simulink model "PMSM_Drehstrom_Regelung"  (R2014b)
settings: Solver=ode4  StartTime=0.0  StopTime=5  FixedStep=1e-6  RelTol=1e-3
undefined symbols (not defined in the file): J, Ld, Lq, n_soll, p, Psi_pm, R1
libraries: simulink x2
settings Model: Creator=benjamin  LastModifiedBy=Benji

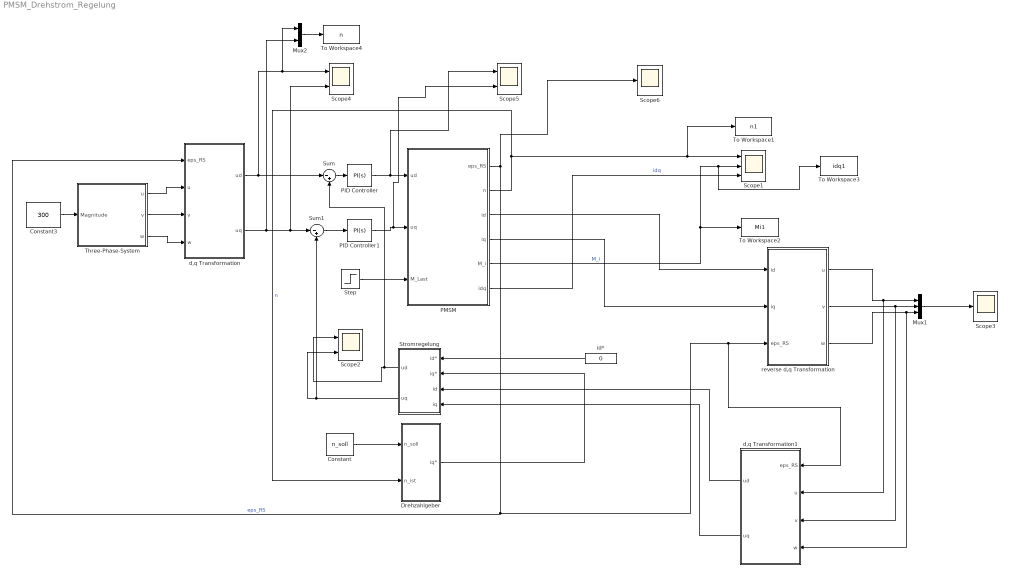
== system PMSM_Drehstrom_Regelung ==
  Constant : Constant  Value=n_soll
  Constant3 : Constant  Value=300
  Drehzahlgeber : Subsystem
  Mux1 : Mux  Inputs=3
  Mux2 : Mux  Inputs=2
  PID Controller : simulink/Continuous/PID Controller  Controller=PI  TimeDomain=Continuous-time  SampleTime=-1  IntegratorMethod=Forward Euler  FilterMethod=Forward Euler  Form=Parallel  P=10  I=1  D=0  N=100  InitialConditionSource=internal  InitialConditionForIntegrator=0  InitialConditionForFilter=0  ExternalReset=none  LimitOutput=off  UpperSaturationLimit=inf  LowerSaturationLimit=-inf  LinearizeAsGain=on  AntiWindupMode=none  Kb=1  TrackingMode=off  Kt=1  PParamMin=[]  PParamMax=[]  IParamMin=[]  IParamMax=[]  DParamMin=[]  DParamMax=[]  NParamMin=[]  NParamMax=[]  KbParamMin=[]  KbParamMax=[]  KtParamMin=[]  KtParamMax=[]  POutMin=[]  POutMax=[]  IOutMin=[]  IOutMax=[]  DOutMin=[]  DOutMax=[]  NOutMin=[]  NOutMax=[]  KbOutMin=[]  KbOutMax=[]  KtOutMin=[]  KtOutMax=[]  IntegratorOutMin=[]  IntegratorOutMax=[]  FilterOutMin=[]  FilterOutMax=[]  SumOutMin=[]  SumOutMax=[]  SumI1OutMin=[]  SumI1OutMax=[]  SumI2OutMin=[]  SumI2OutMax=[]  SumI3OutMin=[]  SumI3OutMax=[]  SumDOutMin=[]  SumDOutMax=[]  SaturationOutMin=[]  SaturationOutMax=[]  IntegratorContinuousStateAttributes=''  IntegratorStateMustResolveToSignalObject=off  IntegratorRTWStateStorageClass=Auto  FilterContinuousStateAttributes=''  FilterStateMustResolveToSignalObject=off  FilterRTWStateStorageClass=Auto  DifferentiatorICPrevScaledInput=0  DifferentiatorOutMin=[]  DifferentiatorOutMax=[]  UseFilter=on
  PID Controller1 : simulink/Continuous/PID Controller  Controller=PI  TimeDomain=Continuous-time  SampleTime=-1  IntegratorMethod=Forward Euler  FilterMethod=Forward Euler  Form=Parallel  P=10  I=1  D=0  N=100  InitialConditionSource=internal  InitialConditionForIntegrator=0  InitialConditionForFilter=0  ExternalReset=none  LimitOutput=off  UpperSaturationLimit=inf  LowerSaturationLimit=-inf  LinearizeAsGain=on  AntiWindupMode=none  Kb=1  TrackingMode=off  Kt=1  PParamMin=[]  PParamMax=[]  IParamMin=[]  IParamMax=[]  DParamMin=[]  DParamMax=[]  NParamMin=[]  NParamMax=[]  KbParamMin=[]  KbParamMax=[]  KtParamMin=[]  KtParamMax=[]  POutMin=[]  POutMax=[]  IOutMin=[]  IOutMax=[]  DOutMin=[]  DOutMax=[]  NOutMin=[]  NOutMax=[]  KbOutMin=[]  KbOutMax=[]  KtOutMin=[]  KtOutMax=[]  IntegratorOutMin=[]  IntegratorOutMax=[]  FilterOutMin=[]  FilterOutMax=[]  SumOutMin=[]  SumOutMax=[]  SumI1OutMin=[]  SumI1OutMax=[]  SumI2OutMin=[]  SumI2OutMax=[]  SumI3OutMin=[]  SumI3OutMax=[]  SumDOutMin=[]  SumDOutMax=[]  SaturationOutMin=[]  SaturationOutMax=[]  IntegratorContinuousStateAttributes=''  IntegratorStateMustResolveToSignalObject=off  IntegratorRTWStateStorageClass=Auto  FilterContinuousStateAttributes=''  FilterStateMustResolveToSignalObject=off  FilterRTWStateStorageClass=Auto  DifferentiatorICPrevScaledInput=0  DifferentiatorOutMin=[]  DifferentiatorOutMax=[]  UseFilter=on
  PMSM : Subsystem
  Scope1 : Scope  NumInputPorts=3
      settings: TimeRange=0.112043795620438  YMin=0~-1000~-4000  YMax=5000~2500~6000  SaveName=ScopeData3
  Scope2 : Scope  NumInputPorts=2
      settings: TimeRange=0.2  YMin=-25000~-400  YMax=20000~400  SaveName=ScopeData2
  Scope3 : Scope
      settings: TimeRange=0.02  YMin=0  YMax=5000  SaveName=ScopeData4
  Scope4 : Scope  NumInputPorts=2
      settings: TimeRange=0.2  YMin=-25000~-400  YMax=20000~400  SaveName=ScopeData5
  Scope5 : Scope  NumInputPorts=2
      settings: TimeRange=0.2  YMin=-25000~-400  YMax=20000~400  SaveName=ScopeData6
  Scope6 : Scope
      settings: TimeRange=0.02  YMin=0  YMax=5000  SaveName=ScopeData7
  Step : Step  Time=0.08  After=30  SampleTime=0
  Stromregelung : Subsystem
  Sum : Sum  Inputs=|-+
  Sum1 : Sum  Inputs=|-+
  Three-Phase-System : Subsystem
  To Workspace1 : ToWorkspace  VariableName=n1  SaveFormat=Timeseries  SampleTime=-1
  To Workspace2 : ToWorkspace  VariableName=Mi1  SaveFormat=Timeseries  SampleTime=-1
  To Workspace3 : ToWorkspace  VariableName=idq1  SaveFormat=Timeseries  SampleTime=-1
  To Workspace4 : ToWorkspace  VariableName=n  SaveFormat=Timeseries  SampleTime=-1
  d,q Transformation : Subsystem
  d,q Transformation1 : Subsystem
  id* : Constant  Value=0
  reverse d,q Transformation : Subsystem
  wires:
  id*/1 -> Stromregelung/1(id*)
  Drehzahlgeber/1(iq*) -> Stromregelung/2(iq*)
  Constant/1 -> Drehzahlgeber/1(n_soll)
  PMSM/2(n) -> To Workspace1/1, Scope1/1, Drehzahlgeber/2(n_ist)  "n"
  PMSM/6(idq) -> Scope1/3  "idq"
  Step/1 -> PMSM/3(M_Last)
  Stromregelung/1(ud) -> Sum/2, Scope2/1
  Stromregelung/2(uq) -> Sum1/2, Scope2/2
  Constant3/1 -> Three-Phase-System/1(Magnitude)
  Three-Phase-System/1(u) -> d,q Transformation/2(u)
  Three-Phase-System/2(v) -> d,q Transformation/3(v)
  Three-Phase-System/3(w) -> d,q Transformation/4(w)
  PMSM/1(eps_RS) -> d,q Transformation1/1(eps_RS), reverse d,q Transformation/3(eps_RS), d,q Transformation/1(eps_RS), Scope6/1  "eps_RS"
  PMSM/3(id) -> reverse d,q Transformation/1(id)
  PMSM/4(iq) -> reverse d,q Transformation/2(iq)
  reverse d,q Transformation/1(u) -> d,q Transformation1/2(u), Mux1/1
  reverse d,q Transformation/2(v) -> Mux1/2, d,q Transformation1/3(v)
  reverse d,q Transformation/3(w) -> d,q Transformation1/4(w), Mux1/3
  Mux1/1 -> Scope3/1
  PMSM/5(M_i) -> To Workspace2/1, To Workspace3/1, Scope1/2  "M_i"
  d,q Transformation/1(ud) -> Mux2/1, Scope4/1, Sum/1
  d,q Transformation/2(uq) -> Mux2/2, Scope4/2, Sum1/1
  Sum/1 -> PID Controller/1
  PID Controller/1 -> Scope5/1, PMSM/1("ud ")
  Sum1/1 -> PID Controller1/1
  PID Controller1/1 -> Scope5/2, PMSM/2(uq)
  d,q Transformation1/1(ud) -> Stromregelung/3(id)
  d,q Transformation1/2(uq) -> Stromregelung/4(iq)
  Mux2/1 -> To Workspace4/1

== system PMSM_Drehstrom_Regelung/Drehzahlgeber ==
  n_soll : Inport
  n_ist : Inport  Port=2
  Gain : Gain  Gain=10
  Gain1 : Gain  Gain=2
  Integrator : Integrator
  Sum : Sum  Inputs=|+-
  Sum1 : Sum  Inputs=|++
  iq* : Outport
  wires:
  n_soll/1 -> Sum/1
  n_ist/1 -> Sum/2
  Sum/1 -> Gain1/1, Gain/1
  Gain/1 -> Sum1/1
  Gain1/1 -> Integrator/1
  Integrator/1 -> Sum1/2
  Sum1/1 -> iq*/1

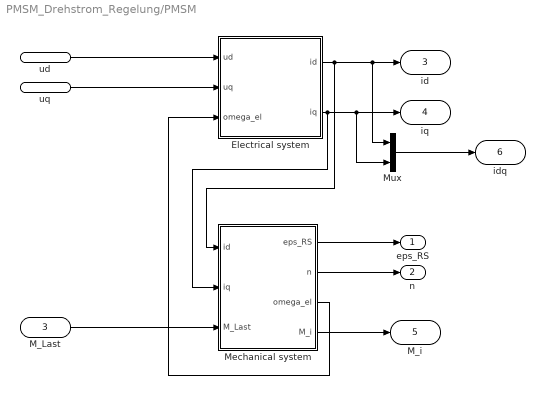
== system PMSM_Drehstrom_Regelung/PMSM ==
  "ud " : Inport
  uq : Inport  Port=2
  M_Last : Inport  Port=3
  Electrical system : Subsystem
  Mechanical system : Subsystem
  Mux : Mux  Inputs=2
  eps_RS : Outport
  n : Outport  Port=2
  id : Outport  Port=3
  iq : Outport  Port=4
  M_i : Outport  Port=5
  idq : Outport  Port=6
  wires:
  Electrical system/1(id) -> Mux/1, id/1, Mechanical system/1(id)
  Electrical system/2(iq) -> Mux/2, iq/1, Mechanical system/2(iq)
  Mechanical system/3(omega_el) -> Electrical system/3(omega_el)
  Mechanical system/1(eps_RS) -> eps_RS/1
  Mechanical system/2(n) -> n/1
  Mechanical system/4(M_i) -> M_i/1
  M_Last/1 -> Mechanical system/3(M_Last)
  uq/1 -> Electrical system/2(uq)
  "ud "/1 -> Electrical system/1(ud)
  Mux/1 -> idq/1

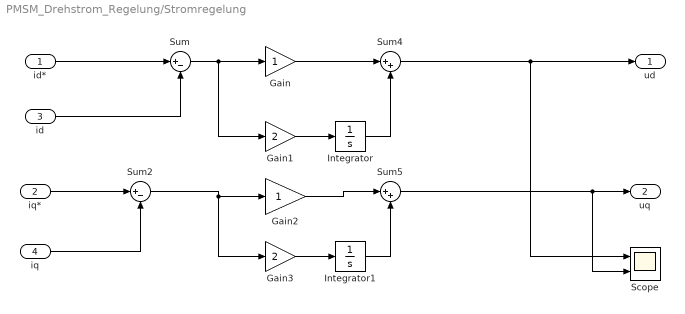
== system PMSM_Drehstrom_Regelung/Stromregelung ==
  id* : Inport
  iq* : Inport  Port=2
  id : Inport  Port=3
  iq : Inport  Port=4
  Gain : Gain
  Gain1 : Gain  Gain=2
  Gain2 : Gain
  Gain3 : Gain  Gain=2
  Integrator : Integrator
  Integrator1 : Integrator
  Scope : Scope  NumInputPorts=2
      settings: TimeRange=5  YMin=-1.3~-5  YMax=0~5
  Sum : Sum  Inputs=|+-
  Sum2 : Sum  Inputs=|+-
  Sum4 : Sum  Inputs=|++
  Sum5 : Sum  Inputs=|++
  ud : Outport
  uq : Outport  Port=2
  wires:
  Sum5/1 -> Scope/2, uq/1
  iq*/1 -> Sum2/1
  id*/1 -> Sum/1
  id/1 -> Sum/2
  iq/1 -> Sum2/2
  Sum4/1 -> ud/1, Scope/1
  Sum/1 -> Gain1/1, Gain/1
  Gain/1 -> Sum4/1
  Gain1/1 -> Integrator/1
  Integrator/1 -> Sum4/2
  Sum2/1 -> Gain3/1, Gain2/1
  Gain2/1 -> Sum5/1
  Gain3/1 -> Integrator1/1
  Integrator1/1 -> Sum5/2

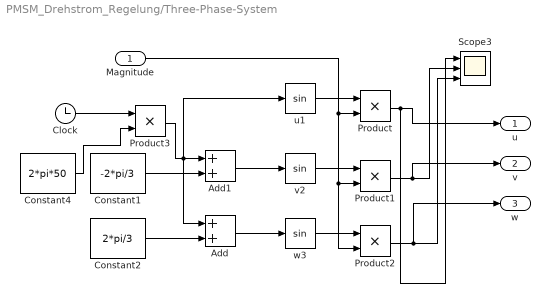
== system PMSM_Drehstrom_Regelung/Three-Phase-System ==
  Magnitude : Inport
  Add : Sum
  Add1 : Sum
  Clock : Clock
  Constant1 : Constant  Value=-2*pi/3
  Constant2 : Constant  Value=2*pi/3
  Constant4 : Constant  Value=2*pi*50
  Product{,1..3} (4 alike) : Product
  Scope3 : Scope  NumInputPorts=3
      settings: YMin=-5~-5~-5  YMax=5~5~5
  u1 : Trigonometry
  v2 : Trigonometry
  w3 : Trigonometry
  u : Outport
  v : Outport  Port=2
  w : Outport  Port=3
  wires:
  Constant2/1 -> Add/2
  Add/1 -> w3/1
  Add1/1 -> v2/1
  Constant1/1 -> Add1/2
  Product2/1 -> w/1, Scope3/3
  Product/1 -> u/1, Scope3/1
  w3/1 -> Product2/1
  Product3/1 -> Add/1, Add1/1, u1/1
  Clock/1 -> Product3/1
  Product1/1 -> v/1, Scope3/2
  Constant4/1 -> Product3/2
  Magnitude/1 -> Product2/2, Product1/2, Product/2
  u1/1 -> Product/1
  v2/1 -> Product1/1

== system PMSM_Drehstrom_Regelung/d,q Transformation ==
  eps_RS : Inport
  u : Inport  Port=2
  v : Inport  Port=3
  w : Inport  Port=4
  Clarke Transformation : Subsystem
  Park Transformation : Subsystem
  ud : Outport
  uq : Outport  Port=2
  wires:
  eps_RS/1 -> Park Transformation/3(epsilonRS)
  Clarke Transformation/1(alpha) -> Park Transformation/1(alpha)
  Clarke Transformation/2(beta) -> Park Transformation/2(beta)
  Park Transformation/1(d) -> ud/1
  Park Transformation/2(q) -> uq/1
  v/1 -> Clarke Transformation/2(v)
  u/1 -> Clarke Transformation/1(u)
  w/1 -> Clarke Transformation/3(w)

== system PMSM_Drehstrom_Regelung/d,q Transformation1 ==
  eps_RS : Inport
  u : Inport  Port=2
  v : Inport  Port=3
  w : Inport  Port=4
  Clarke Transformation : Subsystem
  Park Transformation : Subsystem
  ud : Outport
  uq : Outport  Port=2
  wires:
  eps_RS/1 -> Park Transformation/3(epsilonRS)
  Clarke Transformation/1(alpha) -> Park Transformation/1(alpha)
  Clarke Transformation/2(beta) -> Park Transformation/2(beta)
  Park Transformation/1(d) -> ud/1
  Park Transformation/2(q) -> uq/1
  v/1 -> Clarke Transformation/2(v)
  u/1 -> Clarke Transformation/1(u)
  w/1 -> Clarke Transformation/3(w)

== system PMSM_Drehstrom_Regelung/reverse d,q Transformation ==
  id : Inport
  iq : Inport  Port=2
  eps_RS : Inport  Port=3
  inverse Clarke Transformation : Subsystem
  inverse Park Transformation : Subsystem
  u : Outport
  v : Outport  Port=2
  w : Outport  Port=3
  wires:
  inverse Clarke Transformation/2(iv) -> v/1
  id/1 -> inverse Park Transformation/1(d)
  inverse Clarke Transformation/1(iu) -> u/1
  iq/1 -> inverse Park Transformation/2(q)
  inverse Clarke Transformation/3(iw) -> w/1
  eps_RS/1 -> inverse Park Transformation/3(epsilonRS)
  inverse Park Transformation/1(alpha) -> inverse Clarke Transformation/1(alpha)
  inverse Park Transformation/2(beta) -> inverse Clarke Transformation/2(beta)

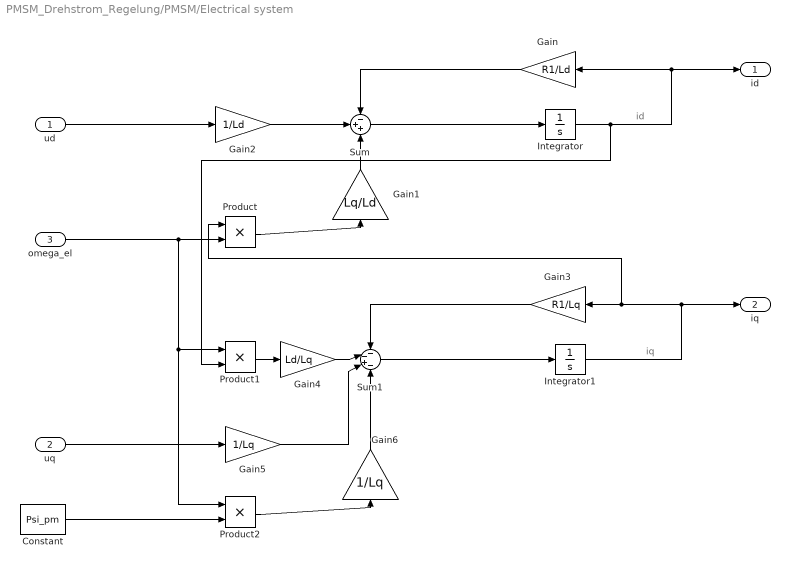
== system PMSM_Drehstrom_Regelung/PMSM/Electrical system ==
  note: id
  note: iq
  ud : Inport
  uq : Inport  Port=2
  omega_el : Inport  Port=3
  Constant : Constant  Value=Psi_pm
  Gain : Gain  Gain=R1/Ld
  Gain1 : Gain  Gain=Lq/Ld
  Gain2 : Gain  Gain=1/Ld
  Gain3 : Gain  Gain=R1/Lq
  Gain4 : Gain  Gain=Ld/Lq
  Gain5 : Gain  Gain=1/Lq
  Gain6 : Gain  Gain=1/Lq
  Integrator : Integrator
  Integrator1 : Integrator
  Product : Product
  Product1 : Product
  Product2 : Product
  Sum : Sum  Inputs=-++
  Sum1 : Sum  Inputs=--+-
  id : Outport
  iq : Outport  Port=2
  wires:
  Sum/1 -> Integrator/1
  Integrator/1 -> Product1/2, Gain/1, id/1
  Gain/1 -> Sum/1
  omega_el/1 -> Product2/1, Product1/1, Product/2
  Gain1/1 -> Sum/3
  Product/1 -> Gain1/1
  ud/1 -> Gain2/1
  Gain2/1 -> Sum/2
  Sum1/1 -> Integrator1/1
  Integrator1/1 -> iq/1, Product/1, Gain3/1
  Gain3/1 -> Sum1/1
  Gain5/1 -> Sum1/3
  Product1/1 -> Gain4/1
  Gain4/1 -> Sum1/2
  uq/1 -> Gain5/1
  Constant/1 -> Product2/2
  Gain6/1 -> Sum1/4
  Product2/1 -> Gain6/1

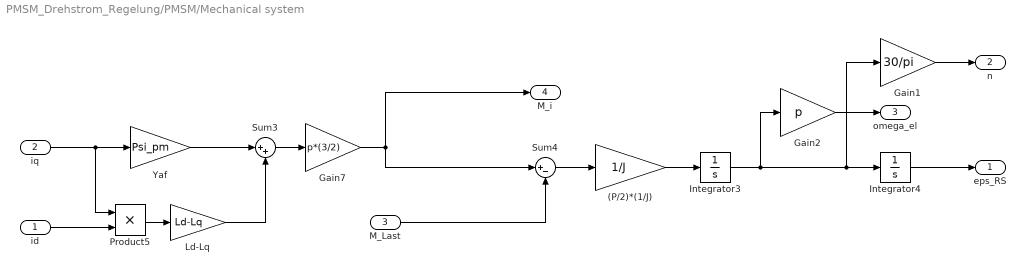
== system PMSM_Drehstrom_Regelung/PMSM/Mechanical system ==
  id : Inport
  iq : Inport  Port=2
  M_Last : Inport  Port=3
  (P/2)*(1/J) : Gain  Gain=1/J
  Gain1 : Gain  Gain=30/pi
  Gain2 : Gain  Gain=p
  Gain7 : Gain  Gain=p*(3/2)
  Integrator3 : Integrator
  Integrator4 : Integrator
  Ld-Lq : Gain  Gain=Ld-Lq
  Product5 : Product  RndMeth=Zero
  Sum3 : Sum  Inputs=|++
  Sum4 : Sum  Inputs=|+-
  Yaf : Gain  Gain=Psi_pm
  eps_RS : Outport
  n : Outport  Port=2
  omega_el : Outport  Port=3
  M_i : Outport  Port=4
  wires:
  Yaf/1 -> Sum3/1
  Sum3/1 -> Gain7/1
  Ld-Lq/1 -> Sum3/2
  Product5/1 -> Ld-Lq/1
  Sum4/1 -> (P/2)*(1/J)/1
  iq/1 -> Product5/1, Yaf/1
  id/1 -> Product5/2
  Gain7/1 -> Sum4/1, M_i/1
  (P/2)*(1/J)/1 -> Integrator3/1
  Integrator4/1 -> eps_RS/1
  Gain1/1 -> n/1
  Integrator3/1 -> Gain1/1, Integrator4/1, Gain2/1
  M_Last/1 -> Sum4/2
  Gain2/1 -> omega_el/1

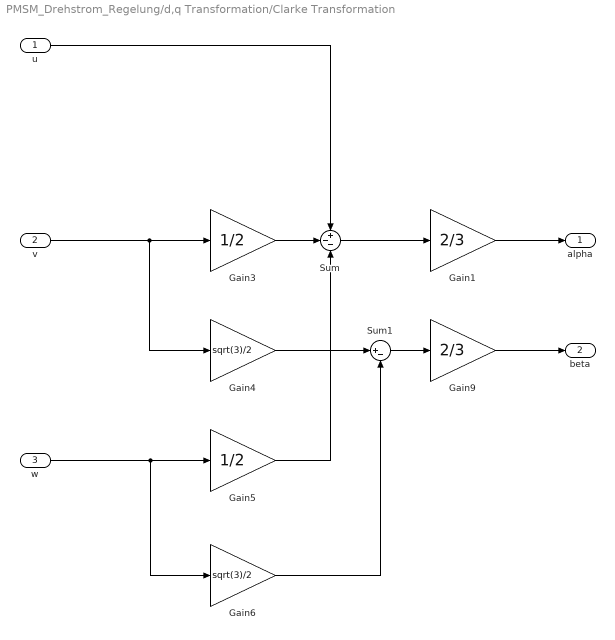
== system PMSM_Drehstrom_Regelung/d,q Transformation/Clarke Transformation ==
  u : Inport
  v : Inport  Port=2
  w : Inport  Port=3
  Gain1 : Gain  Gain=2/3
  Gain3 : Gain  Gain=1/2
  Gain4 : Gain  Gain=sqrt(3)/2
  Gain5 : Gain  Gain=1/2
  Gain6 : Gain  Gain=sqrt(3)/2
  Gain9 : Gain  Gain=2/3
  Sum : Sum  Inputs=+--
  Sum1 : Sum  Inputs=|+-
  alpha : Outport
  beta : Outport  Port=2
  wires:
  Gain5/1 -> Sum/3
  Gain3/1 -> Sum/2
  v/1 -> Gain4/1, Gain3/1
  w/1 -> Gain6/1, Gain5/1
  Gain6/1 -> Sum1/2
  Gain4/1 -> Sum1/1
  Sum/1 -> Gain1/1
  Gain1/1 -> alpha/1
  u/1 -> Sum/1
  Sum1/1 -> Gain9/1
  Gain9/1 -> beta/1

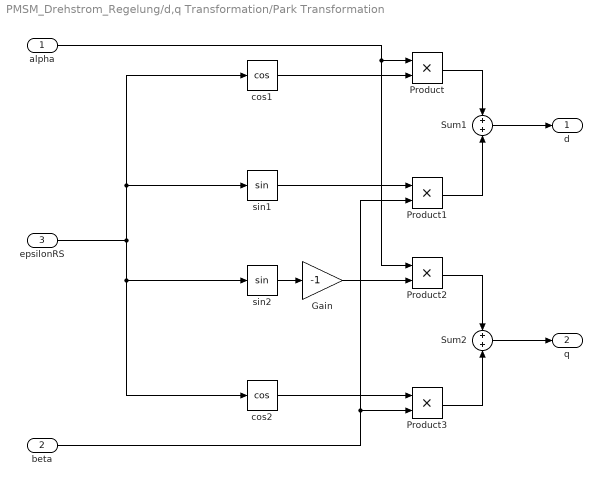
== system PMSM_Drehstrom_Regelung/d,q Transformation/Park Transformation ==
  alpha : Inport
  beta : Inport  Port=2
  epsilonRS : Inport  Port=3
  Gain : Gain  Gain=-1
  Product{,1..3} (4 alike) : Product
  Sum1 : Sum
  Sum2 : Sum
  cos1 : Trigonometry  Operator=cos
  cos2 : Trigonometry  Operator=cos
  sin1 : Trigonometry
  sin2 : Trigonometry
  d : Outport
  q : Outport  Port=2
  wires:
  Sum2/1 -> q/1
  Product2/1 -> Sum2/1
  Product1/1 -> Sum1/2
  epsilonRS/1 -> sin1/1, cos1/1, sin2/1, cos2/1
  cos1/1 -> Product/2
  alpha/1 -> Product2/1, Product/1
  Sum1/1 -> d/1
  cos2/1 -> Product3/1
  beta/1 -> Product3/2, Product1/2
  Product/1 -> Sum1/1
  sin1/1 -> Product1/1
  Product3/1 -> Sum2/2
  sin2/1 -> Gain/1
  Gain/1 -> Product2/2

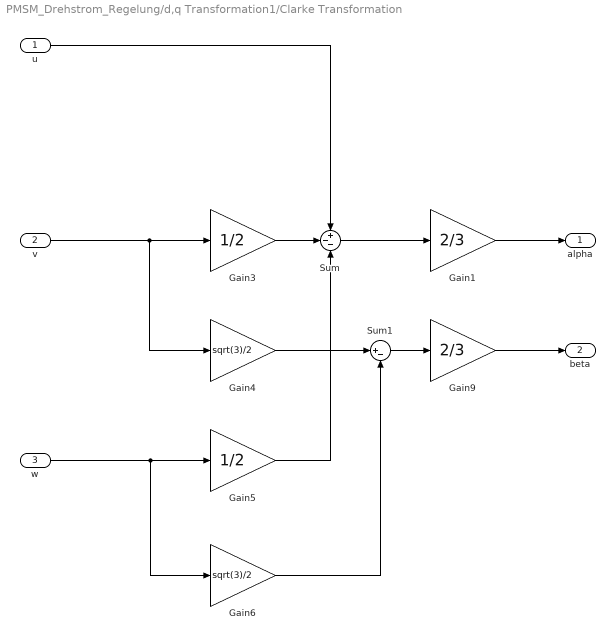
== system PMSM_Drehstrom_Regelung/d,q Transformation1/Clarke Transformation ==
  u : Inport
  v : Inport  Port=2
  w : Inport  Port=3
  Gain1 : Gain  Gain=2/3
  Gain3 : Gain  Gain=1/2
  Gain4 : Gain  Gain=sqrt(3)/2
  Gain5 : Gain  Gain=1/2
  Gain6 : Gain  Gain=sqrt(3)/2
  Gain9 : Gain  Gain=2/3
  Sum : Sum  Inputs=+--
  Sum1 : Sum  Inputs=|+-
  alpha : Outport
  beta : Outport  Port=2
  wires:
  Gain5/1 -> Sum/3
  Gain3/1 -> Sum/2
  v/1 -> Gain4/1, Gain3/1
  w/1 -> Gain6/1, Gain5/1
  Gain6/1 -> Sum1/2
  Gain4/1 -> Sum1/1
  Sum/1 -> Gain1/1
  Gain1/1 -> alpha/1
  u/1 -> Sum/1
  Sum1/1 -> Gain9/1
  Gain9/1 -> beta/1

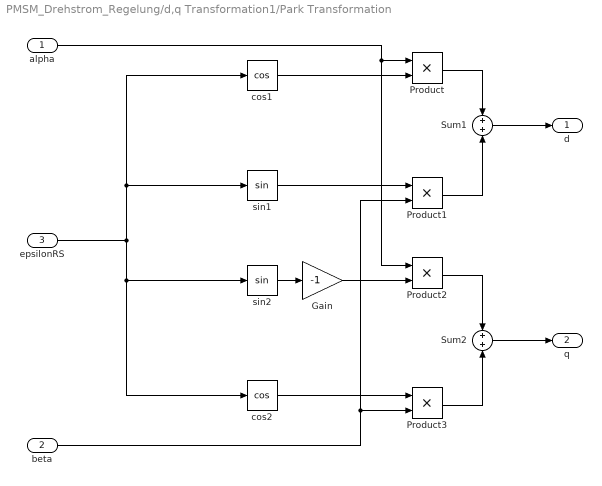
== system PMSM_Drehstrom_Regelung/d,q Transformation1/Park Transformation ==
  alpha : Inport
  beta : Inport  Port=2
  epsilonRS : Inport  Port=3
  Gain : Gain  Gain=-1
  Product{,1..3} (4 alike) : Product
  Sum1 : Sum
  Sum2 : Sum
  cos1 : Trigonometry  Operator=cos
  cos2 : Trigonometry  Operator=cos
  sin1 : Trigonometry
  sin2 : Trigonometry
  d : Outport
  q : Outport  Port=2
  wires:
  Sum2/1 -> q/1
  Product2/1 -> Sum2/1
  Product1/1 -> Sum1/2
  epsilonRS/1 -> sin1/1, cos1/1, sin2/1, cos2/1
  cos1/1 -> Product/2
  alpha/1 -> Product2/1, Product/1
  Sum1/1 -> d/1
  cos2/1 -> Product3/1
  beta/1 -> Product3/2, Product1/2
  Product/1 -> Sum1/1
  sin1/1 -> Product1/1
  Product3/1 -> Sum2/2
  sin2/1 -> Gain/1
  Gain/1 -> Product2/2

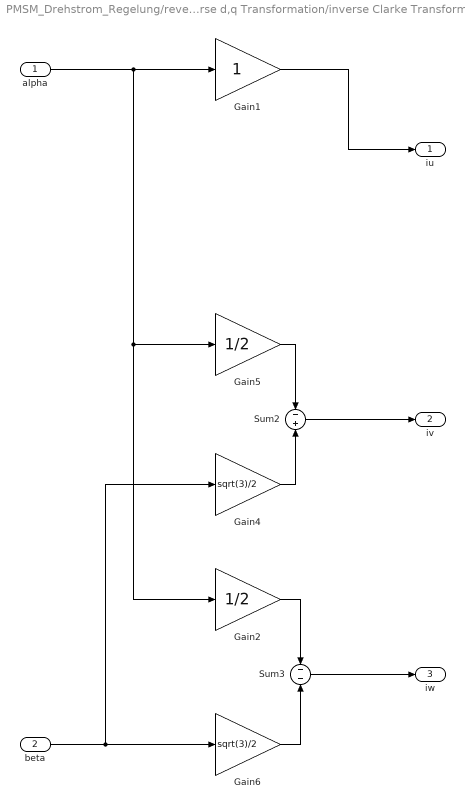
== system PMSM_Drehstrom_Regelung/reverse d,q Transformation/inverse Clarke Transformation ==
  alpha : Inport
  beta : Inport  Port=2
  Gain1 : Gain
  Gain2 : Gain  Gain=1/2
  Gain4 : Gain  Gain=sqrt(3)/2
  Gain5 : Gain  Gain=1/2
  Gain6 : Gain  Gain=sqrt(3)/2
  Sum2 : Sum  Inputs=-+
  Sum3 : Sum  Inputs=--
  iu : Outport
  iv : Outport  Port=2
  iw : Outport  Port=3
  wires:
  Sum2/1 -> iv/1
  beta/1 -> Gain4/1, Gain6/1
  Gain4/1 -> Sum2/2
  Gain5/1 -> Sum2/1
  Gain2/1 -> Sum3/1
  Gain6/1 -> Sum3/2
  alpha/1 -> Gain1/1, Gain2/1, Gain5/1
  Sum3/1 -> iw/1
  Gain1/1 -> iu/1

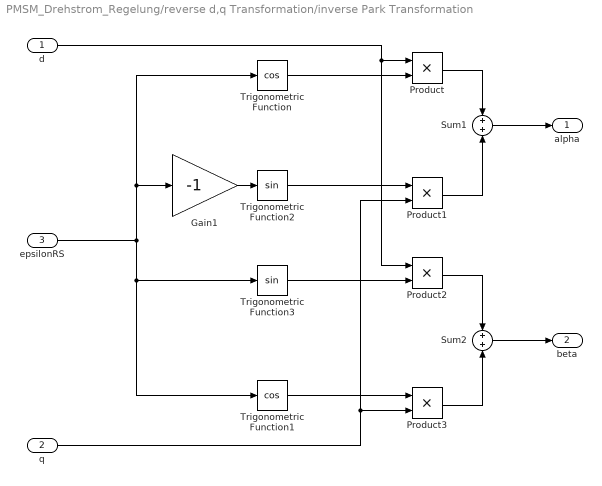
== system PMSM_Drehstrom_Regelung/reverse d,q Transformation/inverse Park Transformation ==
  d : Inport
  q : Inport  Port=2
  epsilonRS : Inport  Port=3
  Gain1 : Gain  Gain=-1
  Product{,1..3} (4 alike) : Product
  Sum1 : Sum
  Sum2 : Sum
  Trigonometric Function : Trigonometry  Operator=cos
  Trigonometric Function1 : Trigonometry  Operator=cos
  Trigonometric Function2 : Trigonometry
  Trigonometric Function3 : Trigonometry
  alpha : Outport
  beta : Outport  Port=2
  wires:
  Sum2/1 -> beta/1
  Product2/1 -> Sum2/1
  Product1/1 -> Sum1/2
  epsilonRS/1 -> Gain1/1, Trigonometric Function/1, Trigonometric Function3/1, Trigonometric Function1/1
  Trigonometric Function/1 -> Product/2
  d/1 -> Product2/1, Product/1
  Sum1/1 -> alpha/1
  Trigonometric Function1/1 -> Product3/1
  q/1 -> Product3/2, Product1/2
  Product/1 -> Sum1/1
  Trigonometric Function2/1 -> Product1/1
  Trigonometric Function3/1 -> Product2/2
  Product3/1 -> Sum2/2
  Gain1/1 -> Trigonometric Function2/1
